simulink model "VFlexP_small"  (R2026a)
settings: Solver=ode23tb  StopTime=2  FixedStep=5e-5
model workspace (MAT data in the model file):
  DCop_DCBUCK : object (value not decoded)
  Grid_CCVSC_idx = [2; 3; 4; 5; 6; 7; 8; 9; 10; 11; 12]
  Grid_CCVSCs = 1
  Grid_CCVSCs_buses = 1
  Grid_CCVSCs_toM = [0 1 0 0 0 0 0 0 0 0 0 0 ... (781 elements, 71x11)]
  Grid_C_Lines = 0
  Grid_Cbuses = [0.00666666666667 0.00666666666667]
  Grid_DC : object (value not decoded)
  Grid_DCop_DCBUCK : object (value not decoded)
  Grid_DCop_DC_PES : object (value not decoded)
  Grid_DFIGs = 1
  Grid_DFIGs_buses = 1
  Grid_DGs : string (value not decoded)
  Grid_From_buses = 1
  Grid_GFls = 1
  Grid_GFls_buses = 1
  Grid_GFr_idx = 1
  Grid_GFrs = 1
  Grid_GFrs_buses = 1
  Grid_GFrs_toM = [1; 0]
  Grid_IG_idx = 1
  Grid_IGs = 1
  Grid_IGs_buses = 1
  Grid_IGs_toM = [1; 0; 0]
  Grid_L_Lines = 0.05
  Grid_L_Loads = [0 0]
  Grid_Lines_fromM : object (value not decoded)
  Grid_Lines_toM : object (value not decoded)
  Grid_Load_buses = [1; 2]
  Grid_Load_busesDC = []
  Grid_MSGs = 1
  Grid_MSGs_buses = 1
  Grid_Nbuses = 2
  Grid_PQ_gen = 3
  Grid_Ploads = [0.0075 0.0075]
  Grid_PloadsDC = []
  Grid_Ps_lf = 0.51232912
  Grid_Qloads = [0 0]
  Grid_Qs_lf = -0.00723209333333
  Grid_R_Lines = 0.005
  Grid_R_Loads = [2 2]
  Grid_R_Loads_DC = 0
  Grid_Rcf = [150 150]
  Grid_SCs = 1
  Grid_SCs_buses = 1
  Grid_SG_idx = 1
  Grid_SGs = 1
  Grid_SGs_buses = 1
  Grid_SGs_toM = [1; 0]
  Grid_To_buses = 2
  Grid_VCVSC_idx = [1; 2; 3; 4; 5; 6; 7; 8; 9; 10; 11; 12]
  Grid_VCVSCs = 1
  Grid_VCVSCs_buses = [1; 2; 3; 6; 8; 9; 12; 58; 59; 60; 63; 65]
  Grid_VCVSCs_toM = [1 0 0 0 0 0 0 0 0 0 0 0 ... (852 elements, 71x12)]
  Grid_VSM_idx = 2
  Grid_VSMs = 1
  Grid_VSMs_buses = 1
  Grid_VSMs_toM = [0; 1]
  Grid_admitt_matrix = [2.15353135314-19.7953135314i  -1.9801980198+19.801980198i; -1.9801980198+19.801980198i  2.15353135314-19.7953135314i]
  Grid_admitt_matrix_noloads = [1.98686468647-19.7953135314i  -1.9801980198+19.801980198i; -1.9801980198+19.801980198i  1.98686468647-19.7953135314i]
  Grid_bus = [1; 2]
  Grid_busDC_complexity = 1
  Grid_busDC_complexity_PF = 2
  Grid_bus_complexity = [1 1]
  Grid_bus_complexity_PF = [1 1]
  Grid_buses_lf = 1
  Grid_conductance_matrix = 0.00666666666667
  Grid_conductance_matrix_noloads = 0.00666666666667
  Grid_fref : object (value not decoded)
  Grid_gen_static_params : mBase (value not decoded)
  Grid_iPs_lf = 1.95187031336
  Grid_iQs_lf = -138.272551792
  Grid_iadmitt_matrix = [2.88165849328-0.0982918688642i  2.87905051706-0.123273862303i; 2.87905051706-0.123273862303i  2.88165849328-0.0982918688642i]
  Grid_iadmitt_matrix_noloads = [37.5012524798-37.4874983544i  37.4987475202-37.5125016456i; 37.4987475202-37.5125016456i  37.5012524798-37.4874983544i]
  Grid_iconductance_matrix = 150
  Grid_iconductance_matrix_noloads = 150
  Grid_init_OK_bool = 1
  Grid_intconv_PF : object (value not decoded)
  Grid_lf_op : op_report (value not decoded)
  Grid_lineDC_complexity = []
  Grid_lineDC_complexity_PF = []
  Grid_line_complexity = 1
  Grid_line_complexity_PF = 3
  Grid_loadDC_complexity = []
  Grid_loadDC_complexity_PF = []
  Grid_load_complexity = [3 3]
  Grid_load_complexity_PF = [4 4]
  Grid_opDC_CCVSC : object (value not decoded)
  Grid_opDC_VSM : object (value not decoded)
  Grid_opGFr : object (value not decoded)
  Grid_opVCVSC : object (value not decoded)
  Grid_op_CCVSC : object (value not decoded)
  Grid_op_IG : object (value not decoded)
  Grid_op_SG : object (value not decoded)
  Grid_op_VSM : object (value not decoded)
  Grid_shift_lines = 0
  Grid_tap_lines = 1
  Grid_v_buses_mod = [1 1]
  LinsysParamChangeStruct : Param1 (value not decoded)
  Lline = 0.01
  Rline = 1e-05
  linsys : object (value not decoded)
values from neighbouring files (symbols this model uses):
  block_idx = evalin(mdlWks, [bvarname Generators{i} '_idx'])    [fun_init_units_callback.m]
  Fb = areas    [fun_MATPOWER_to_Excel.m]
  Fi = evalin('base', get_param(block, 'Fi'))    [fun_init_GFr.m]    (also in fun_init_intconv_DC_VSM.m)
  Lf = evalin('base', get_param(block, 'Lf'))    [fun_init_GFr.m]    (also in fun_init_intconv_DC_VSM.m)
  Rf = evalin('base', get_param(block, 'Rf'))    [fun_init_GFr.m]    (also in fun_init_intconv_DC_VSM.m)
symbols that are objects in the model workspace (value not decoded): Grid_DCop_DC_PES, Grid_DCop_DCBUCK, Grid_op_CCVSC, Grid_op_IG, Grid_op_SG, Grid_op_VSM, Grid_opDC_CCVSC, Grid_opDC_VSM, Grid_opGFr, Grid_opVCVSC
undefined symbols (not defined in the file or in its folder): block_buses_DC, CCVSC_idx, Cf, costs, costs2, DFIGs_nodes, DiscIntNeverNeededParam, entity, From_nodes, grid_linsys, Grid_op_DFIG, Grid_op_DFIG_PQ, Grid_op_MSG, Grid_op_SC, Grid_op_VCVSC, Hv, initial_states_grid, Kic, Kiv, Kp_theta, Kp_w, Kpc, Kpv, last_send, Lc, m, Matrix_flux_to_i, mD, mp, MSGs_buses, Nbuses_DC, nq, op_VCVSC, Psche, Rc, rkq1, rkq2, SCs_buses, SCs_nodes, sec_control_structure, set_asked, set_DG_up, set_extra_satur, set_sending_cost, SGs_buses, SGs_nodes, Tf, To_nodes, VI_L, VI_R, WOF_Tf, xkq1, xkq2
libraries: simulink x1045, eeGeneralControl x12, eeTransforms x1, sl_discontinuities x1
(part 4 of 50)

== system VFlexP_small/Grid/Loadflow/Generators ==
  vd : Inport
  vq : Inport  Port=2
  Constant : Constant  Value=Ps_lf  VectorParams1D=off
  E^* : Integrator  InitialCondition=ones(1, length(buses_lf))  UpperSaturationLimit=1.2  LowerSaturationLimit=0.8
  Gain : Gain  Gain=double(PQ_gen==1)
  Gain1 : Gain  Gain=-1
  Gain10 : Gain  Gain=1e-3
  Gain11 : Gain  Gain=double(PQ_gen==3)
  Gain12 : Gain  Gain=double(PQ_gen~=3)
  Gain2 : Gain  Gain=double(PQ_gen~=1)
  Gain3 : Gain
  Gain4 : Gain
  Gain5 : Gain  Gain=double(PQ_gen==1)
  Gain6 : Gain  Gain=2*pi*50
  Gain7 : Gain  Gain=double(PQ_gen~=1)
  Gain8 : Gain  Gain=-1
  Gain9 : Gain  Gain=1e-3
  Gen_To : MATLAB Function  TreatAsAtomicUnit=on
  Gen_To1 : MATLAB Function  TreatAsAtomicUnit=on
  One1 : Constant  Value=Qs_lf  VectorParams1D=off  OutDataTypeStr=Inherit: Inherit via back propagation
  One3 : Constant  Value=v_buses_mod(buses_lf)  VectorParams1D=off  OutDataTypeStr=Inherit: Inherit via back propagation
  P : Gain  Gain=iPs_lf
  PC : Subsystem
  Q : Gain  Gain=iQs_lf
  RL out : Subsystem  Variant=on  VariantControlMode=label  LabelModeActiveChoice=dynamic  mask{dynamic=Dynamic, R=0.01, L=0.1, fbase=50}
      mask prompts: dynamic "Dynamic behavior"; R "Series resistance (p.u.)"; L "Inductance (p.u.)"; fbase "Base frequency (Hz)"
      mask init:
      | omegab = 2*pi*fbase;
      | invL = 1./L;
      | vssBlk = gcb;
      | switch dynamic
      |     case "Static"
      |         set_param(vssBlk, 'LabelModeActiveChoice', 'static');
      |     case "Dynamic"
      |         set_param(vssBlk, 'LabelModeActiveChoice', 'dynamic');
      |     case "Static omega"
      |         set_param(vssBlk, 'LabelModeActiveChoice', 'static_omega');
      | end
      mask TypeOptions dynamic: Static | Dynamic | Static omega
  Real-Imag to Complex : RealImagToComplex
  Reference frame transform1 : Subsystem
  Reference frame transform2 : Subsystem
  Reference frame transform3 : Subsystem
  Sum : Sum  Inputs=|--
  Sum1 : Sum  Inputs=|+-
  Sum2 : Sum  Inputs=-+|
  Sum3 : Sum  Inputs=|++
  Sum4 : Sum  Inputs=-+|
  Sum5 : Sum  Inputs=|--
  Sum6 : Sum  Inputs=|+-
  Sum7 : Sum  Inputs=|-+
  Sum8 : Sum  Inputs=|++
  Sum9 : Sum  Inputs=|++
  Zero : Constant  Value=0  OutDataTypeStr=Inherit: Inherit via back propagation
  \omega^* : Integrator  InitialCondition=ones(1, length(buses_lf))
  frame : Integrator  InitialCondition=zeros(1, length(buses_lf))  IgnoreLimit=on
  select_vd : Selector  InputPortWidth=Nbuses  IndexOptions=Index vector (dialog)  Indices=buses_lf  OutputSizes=1
  select_vq : Selector  InputPortWidth=Nbuses  IndexOptions=Index vector (dialog)  Indices=buses_lf  OutputSizes=1
  v : ComplexToMagnitudeAngle  Output=Magnitude
  i_d : Outport
  i_q : Outport  Port=2
  wires:
  [omega] -> Sum2/2
  Sum4/1 -> Gain9/1
  [omega] -> Sum1/1  "omega"
  [P_f] -> Sum4/2
  Sum/1 -> Gain3/1
  [P_s_to_follow] -> Sum4/1
  Gain9/1 -> Sum/2
  \omega^*/1 -> PC/3(omegaref)
  [omega_ref] -> Sum1/2
  E^*/1 -> PC/4(Eref)
  [v_to_follow] -> Sum6/2
  Sum6/1 -> Sum5/1
  Sum5/1 -> Gain4/1
  Sum7/1 -> Gain10/1
  [Q_s_to_follow] -> Sum7/1
  [vod] -> Real-Imag to Complex/1
  [Q_f] -> Sum7/2
  Gain10/1 -> Sum5/2
  PC/2(Out2) -> [vodref]
  PC/1(Out1) -> [omega]
  Q/1 -> [Q_s]
  P/1 -> [P_s]
  PC/4(Q_f) -> Q/1, [Q_f]
  PC/3(P_f) -> P/1, [P_f]
  [iod] -> PC/2(iodi)
  [theta] -> Reference frame transform3/2(theta)
  select_vd/1 -> Reference frame transform2/1(in_d), RL out/2(v_out_d)
  select_vq/1 -> Reference frame transform2/3(in_q), RL out/4(v_out_q)
  [voq] -> PC/6(voq)
  Gain1/1 -> Reference frame transform1/2(theta)
  [ioq] -> PC/1(ioq)
  Reference frame transform1/1(out_d) -> [iod]
  Reference frame transform3/1(out_d) -> RL out/1(v_in_d)
  Zero/1 -> Reference frame transform3/3(in_q)
  RL out/2(iq) -> Gen_To1/1(u), Reference frame transform1/3(in_q)
  [theta] -> Gain1/1
  Reference frame transform1/2(out_q) -> [ioq]
  Gain6/1 -> frame/1
  Reference frame transform3/2(out_q) -> RL out/3(v_in_q)
  [vod] -> PC/5(vodi)
  [vodref] -> Reference frame transform3/1(in_d)
  Gen_To/1(y) -> i_d/1
  Gen_To1/1(y) -> i_q/1
  RL out/1(id) -> Gen_To/1(u), Reference frame transform1/1(in_d)
  [omega_ref] -> Sum2/1  "ref_omega"
  Sum2/1 -> Gain6/1
  vd/1 -> select_vd/1
  vq/1 -> select_vq/1
  [P_f] -> Gain11/1
  frame/1 -> [theta]
  Constant/1 -> Gain12/1
  Sum1/1 -> Sum/1
  Gain/1 -> Sum3/1
  Gain2/1 -> Sum3/2
  Sum3/1 -> [v_to_follow]
  One3/1 -> Gain2/1
  v/1 -> Gain/1, Sum6/1
  Gain7/1 -> Sum8/2
  Gain5/1 -> Sum8/1
  [Q_f] -> Gain7/1
  One1/1 -> Gain5/1
  Sum8/1 -> [Q_s_to_follow]
  Gain4/1 -> E^*/1
  Gain3/1 -> \omega^*/1
  [theta] -> Gain8/1
  Gain8/1 -> Reference frame transform2/2(theta)
  Reference frame transform2/2(out_q) -> [voq]
  Reference frame transform2/1(out_d) -> [vod]
  [voq] -> Real-Imag to Complex/2
  Real-Imag to Complex/1 -> v/1
  Sum9/1 -> [P_s_to_follow]
  Gain11/1 -> Sum9/1
  Gain12/1 -> Sum9/2

== system VFlexP_small/Grid/Loadflow/Grid ==
  note: 1) Add Subsystem or Model blocks as valid variant choices.
      | 2) You cannot connect blocks at this level. At simulation, connectivity is automatically
      | determined, based on the active variant and port name matching.
  id_in : Inport
  iq_in : Inport  Port=2
  id_out : Inport  Port=3
  iq_out : Inport  Port=4
  Dynamic : Subsystem  VariantControl=Dynamic
  Static : Subsystem  VariantControl=Static
  vd : Outport
  vq : Outport  Port=2

== system VFlexP_small/Grid/Loadflow/Loads ==
  vd : Inport
  vq : Inport  Port=2
  PQ : Subsystem  VariantControl=PQ
  Sum : Sum  Inputs=|+++++
  Sum1 : Sum  Inputs=|+++++
  dynamic : Subsystem  Commented=on  VariantControl=dynamic
  dynamic PQ : Subsystem  Commented=on  VariantControl=PQ
  static : Subsystem  Commented=on  VariantControl=static
  static omega : Subsystem  Commented=on  VariantControl=static_omega
  id : Outport
  iq : Outport  Port=2
  wires:
  dynamic/1(id) -> Sum/1
  vq/1 -> dynamic PQ/2(v_in_q), PQ/2(v_in_q), static omega/2(v_in_q), static/2(v_in_q), dynamic/2(v_in_q)
  PQ/2(iq) -> Sum1/4
  dynamic PQ/2(iq) -> Sum1/5
  vd/1 -> dynamic PQ/1(v_in_d), PQ/1(v_in_d), static omega/1(v_in_d), static/1(v_in_d), dynamic/1(v_in_d)
  static omega/1(id) -> Sum/3
  Sum/1 -> id/1  "id"
  static omega/2(iq) -> Sum1/3
  dynamic PQ/1(id) -> Sum/5
  static/2(iq) -> Sum1/2
  Sum1/1 -> iq/1  "iq"
  dynamic/2(iq) -> Sum1/1
  PQ/1(id) -> Sum/4
  static/1(id) -> Sum/2

== system VFlexP_small/Grid/Loadflow/to_all_Nodes ==
  In1 : Inport
  Assignment : Assignment  DiagnosticForDimensions=Warning  IndexOptions=Index vector (dialog)  Indices=Load_buses  OutputSizes=1
  Zero : Constant  Value=zeros(1,Nbuses)  VectorParams1D=off  OutDataTypeStr=Inherit: Inherit via back propagation
  id_out : Outport
  wires:
  Zero/1 -> Assignment/1
  In1/1 -> Assignment/2
  Assignment/1 -> id_out/1

== system VFlexP_small/Grid/Loadflow/to_all_Nodes1 ==
  In1 : Inport
  Assignment : Assignment  DiagnosticForDimensions=Warning  IndexOptions=Index vector (dialog)  Indices=Load_buses  OutputSizes=1
  Zero : Constant  Value=zeros(1,Nbuses)  VectorParams1D=off  OutDataTypeStr=Inherit: Inherit via back propagation
  iq_out : Outport
  wires:
  Assignment/1 -> iq_out/1
  In1/1 -> Assignment/2
  Zero/1 -> Assignment/1

== system VFlexP_small/Grid/Dynamic/DCAC converters/DC_CCVSC ==
  note: port number 2
  note: do not rename this block, conditions to initialise the generator from PF result are set on this block's output
  vac : Inport
  vdc : Inport  Port=2
  Abs : Abs  SaturateOnIntegerOverflow=off
  CC : Subsystem  Variant=on  VariantControlMode=label  LabelModeActiveChoice=dynamic
  Cast To Double : DataTypeConversion  OutDataTypeStr=double  SaturateOnIntegerOverflow=off  RndMeth=Floor
  Compare To Constant : simulink/Logic and Bit Operations/Compare To Constant  relop===  const=2  OutDataTypeStr=boolean
  Complex to Magnitude-Angle : ComplexToMagnitudeAngle  Output=Angle
  Constant : Constant  Value=zeros(1, length(block_buses))  VectorParams1D=off
  Constant1 : Constant  Value=dparams.alpha1  VectorParams1D=off
  Constant2 : Constant  Value=dparams.type  VectorParams1D=off
  Constant3 : Constant  Value=DC.v(block_DC_buses)  VectorParams1D=off
  Divide : Product  Inputs=*/
  For Each Subsystem : Subsystem  TreatAsAtomicUnit=on
  Gain : Gain  Gain=-1
  Gain1 : Gain  Gain=dparams.alpha2
  Gain10 : Gain  Gain=-1
  Gain2 : Gain  Gain=dparams.alpha3
  Gain5 : Gain  Gain=0.5
  Gain8 : Gain  Gain=10
  Gain9 : Gain
  Gsw : Constant  Value=dparams.Gsw.*(dparams.alpha1 == 0 & dparams.alpha2 == 0 & dparams.alpha3 == 0)  VectorParams1D=off
  I : Integrator  InitialCondition=Grid_opDC_CCVSC.P
  LPF_d : Subsystem
  LPF_q : Subsystem
  Matrix Concatenate1 : Concatenate  NumInputs=3  Mode=Multidimensional array
  One : Constant  OutDataTypeStr=Inherit: Inherit via back propagation
  P : Integrator  InitialCondition=Grid_opDC_CCVSC.P
  PC : Subsystem
      settings: PortSchema="{\"entries\":[{\"content\":{\"sides\":[{\"content\":{\"connectorIds\":[\"In1\",\"In2\",\"In3\",\"In4\"]},\"type\":\"ConnectorPlacement.EquallySpacedRectSide\",\"uuid\":\"7748ce6f-2dcc-431c-b3ea-0be9c3088b1d\"},{\"content\":{\"connectorIds\":[\"In5\",\"Out1\",\"Out2\"],\"side\":\"RIGHT\"},\"type\":\"ConnectorPlacement.EquallySpacedRectSide\",\"uuid\":\"af86fd8d-043b-4d20-8ee8-e7a977d706a8\"},{\"content\":{\"side\":\"TOP\"},\"type\":\"ConnectorPlacement.EquallySpacedRectSide\",\"uuid\":\"807e0dc6-0d59-4ea5-9557-3ccfd29c2ad0\"}]},\"type\":\"ConnectorPlacement.EquallySpacedConnector\",\"uuid\":\"c7fe00c5-0a0a-4038-b7ac-e659fb2aa4a7\"}],\"packageUris\":[\"http://schema.mathworks.com/mf0/Connector/R2020b\"],\"version\":\"1.0\"}"
  PLL : Subsystem  Variant=on  VariantControlMode=label  LabelModeActiveChoice=dynamic
  Product{,1..5,8} (7 alike) : Product
  Product6 : Product  Inputs=3
  Q : Integrator  InitialCondition=Grid_opDC_CCVSC.Q
  Real-Imag to Complex : RealImagToComplex
  Real-Imag to Complex1 : RealImagToComplex
  Reference frame transform3 : Subsystem
  Reference_frame_transform1 : Subsystem
  Scope : Scope
      settings: ActiveDisplayYMinimum=-0.01179  ActiveDisplayYMaximum=0.0098
  Scope1 : Scope
      settings: ActiveDisplayYMinimum=-0.59827  ActiveDisplayYMaximum=0.48453  DataLoggingVariableName=ScopeData2
  Selector : Selector  InputPortWidth=DC.Nbuses  IndexOptions=Index vector (dialog)  Indices=block_DC_buses  OutputSizes=1
  Selector5 : Selector  NumberOfDimensions=2  InputPortWidth=3  IndexOptions=Index vector (dialog),Index vector (dialog)  Indices=1,block_buses  OutputSizes=1,1
  Selector6 : Selector  NumberOfDimensions=2  InputPortWidth=3  IndexOptions=Index vector (dialog),Index vector (dialog)  Indices=2,block_buses  OutputSizes=1,1
  Selector7 : Selector  InputPortWidth=length(fref.ref_units)  IndexOptions=Index vector (dialog)  Indices=block_fref  OutputSizes=1
  Signal Specification1 : SignalSpecification  Dimensions=[3 length(block_buses)]
  State-Space : StateSpace  A=[]  B=[]  C=[]  D=block_DC_toM  InitialCondition=0  ParameterTunability=Optimized
  Sum : Sum  Inputs=|++
  Sum1 : Sum  Inputs=|-+
  Sum2 : Sum  Inputs=|++
  Sum4 : Sum  Inputs=+|+|+
  Sum5 : Sum  Inputs=+|+|+
  Sum6 : Sum  Inputs=|++
  Sum7 : Sum  Inputs=|+-
  Switch : Switch  Criteria=u2 > Threshold  SaturateOnIntegerOverflow=off  InputSameDT=off
  Terminator{,3..5} (4 alike) : Terminator
  Transpose : Math  Operator=transpose
  Transpose1 : Math  Operator=transpose
  connect : Subsystem
  connect1 : Subsystem
      settings: PortSchema="{\"entries\":[{\"content\":{\"sides\":[{\"content\":{\"connectorIds\":[\"In1\",\"In2\"]},\"type\":\"ConnectorPlacement.EquallySpacedRectSide\",\"uuid\":\"6197940c-2174-4524-96b1-99ee20c84056\"},{\"content\":{\"connectorIds\":[\"Out1\",\"Out2\"],\"side\":\"RIGHT\"},\"type\":\"ConnectorPlacement.EquallySpacedRectSide\",\"uuid\":\"9096a550-ff71-4818-a7e7-327a4860b088\"},{\"content\":{\"connectorIds\":[\"In3\"],\"side\":\"TOP\"},\"type\":\"ConnectorPlacement.EquallySpacedRectSide\",\"uuid\":\"d804310e-982f-4fb4-ab62-6be4f27f3ef7\"}]},\"type\":\"ConnectorPlacement.EquallySpacedConnector\",\"uuid\":\"3c08874d-8366-4035-b771-5fa3fbbe507b\"}],\"packageUris\":[\"http://schema.mathworks.com/mf0/Connector/R2020b\"],\"version\":\"1.0\"}"
  trim_output : Subsystem
  iac : Outport
  idc : Outport  Port=2
  wires:
  vac/1 -> Selector5/1, Selector6/1
  Selector6/1 -> [vqout], trim_output/4(vq)
  Selector5/1 -> [vdout], trim_output/3(vd)
  trim_output/4(Out4) -> Terminator5/1
  trim_output/2(Out2) -> Terminator3/1
  trim_output/3(Out3) -> Terminator4/1
  trim_output/1(Out1) -> Terminator/1
  For Each Subsystem/1(Out1) -> iac/1
  Constant/1 -> Matrix Concatenate1/3
  Signal Specification1/1 -> For Each Subsystem/1(In1)
  Matrix Concatenate1/1 -> Signal Specification1/1
  [v_q_PCC] -> Reference frame transform3/3(in_q), Real-Imag to Complex/2  "voq"
  [v_d_PCC] -> Reference frame transform3/1(in_d), Real-Imag to Complex/1  "vod"
  connect/2(iq_real) -> Matrix Concatenate1/2, trim_output/2(iq), [ioq]
  connect/1(id_real) -> Matrix Concatenate1/1, trim_output/1(id), [iod]
  One/1 -> connect/3(connect), connect1/3(connect)
  Cast To Double/1 -> [connected]
  Reference_frame_transform1/1(dout) -> connect/1(id)
  Reference_frame_transform1/2(qout) -> connect/2(iq)
  PLL/2(omega_point) -> [omega], CC/5(omega)  "\\omega CCVSC"
  Complex to Magnitude-Angle/1 -> [voutangle]
  Real-Imag to Complex/1 -> Complex to Magnitude-Angle/1
  [vod] -> CC/3(vod), PC/1(vodi)
  [voq] -> CC/4(voq), PC/2(voq)
  Reference frame transform3/1(out_d) -> [vod]  "v CCVSC"
  [v_q_PCC] -> Product1/1  "voq"
  Sum/1 -> LPF_d/1(In1)
  Sum1/1 -> LPF_q/1(In1)
  [iod] -> Product3/2  "iod"
  [ioq] -> Product2/2  "ioq"
  Product2/1 -> Sum1/1
  Product1/1 -> Sum/2
  Product3/1 -> Sum1/2
  Product/1 -> Sum/1
  LPF_d/1(Out1) -> Scope/1, [P_s]
  LPF_q/1(Out1) -> Scope1/1, [Q_s]
  [v_d_PCC] -> Product/1  "vod"
  [iod] -> Product/2  "iod"
  [ioq] -> Product1/2  "ioq"
  [v_d_PCC] -> Product2/1  "vod"
  [v_q_PCC] -> Product3/1  "voq"
  PC/1(Output) -> CC/1(idref)  "iod"
  PC/2(Output1) -> CC/2(iqref)  "ioq"
  [theta] -> Gain/1
  Gain/1 -> Reference frame transform3/2(theta)
  [theta] -> Reference_frame_transform1/3(theta)
  [voq] -> PLL/2(vq)
  [omega_ref] -> Selector7/1
  PLL/1(theta) -> [theta]
  Reference frame transform3/2(out_q) -> [voq]
  connect/3(connected) -> Cast To Double/1
  Q/1 -> PC/4(vodi2)
  [voutangle] -> PLL/1(voutangle)
  Product4/1 -> Sum2/1
  Product5/1 -> Sum2/2
  connect1/2(iq_real) -> Product5/2, Real-Imag to Complex1/2  "ioq"
  connect1/1(id_real) -> Real-Imag to Complex1/1, Product4/2  "iod"
  CC/3(vid) -> Product4/1
  CC/4(viq) -> Product5/1
  Real-Imag to Complex1/1 -> Abs/1
  Constant1/1 -> Sum4/3
  Gain1/1 -> Sum4/2
  Product8/1 -> Gain2/1
  Gain2/1 -> Sum4/1
  Sum5/1 -> Gain10/1  "Pdc"
  Divide/1 -> Transpose/1  "iDC"
  [vdout] -> [v_d_PCC]
  [vqout] -> [v_q_PCC]
  P/1 -> Switch/3
  Switch/1 -> PC/3(vodi1)
  Constant2/1 -> Compare To Constant/1
  Gain5/1 -> Sum6/1
  I/1 -> Sum6/2
  Gain8/1 -> I/1
  Sum6/1 -> Switch/1
  Constant3/1 -> Sum7/2
  Gain9/1 -> Gain8/1, Gain5/1
  CC/1(idiref) -> connect1/1(id), Reference_frame_transform1/1(din)
  CC/2(iqiref) -> Reference_frame_transform1/2(qin), connect1/2(iq)  "ioq"
  Sum7/1 -> Gain9/1
  Compare To Constant/1 -> Switch/2
  Sum2/1 -> Sum5/2
  Gain10/1 -> Divide/1
  Product6/1 -> Sum5/3
  Abs/1 -> Product8/2, Product8/1, Gain1/1
  Sum4/1 -> Sum5/1
  Gsw/1 -> Product6/1
  State-Space/1 -> Transpose1/1
  Transpose/1 -> State-Space/1
  [vDC] -> Sum7/1
  Selector7/1 -> PC/5(omega), PLL/3(omega)
  Transpose1/1 -> idc/1
  Selector/1 -> Product6/3, Product6/2, [vDC], Divide/2
  vdc/1 -> Selector/1

== system VFlexP_small/Grid/Dynamic/DCAC converters/DC_VCVSC ==
  note: port number 2
  note: do not rename this block, conditions to initialise the generator from PF result are set on this block's output
  vac : Inport
  vdc : Inport  Port=2
  AND : Logic  IconShape=distinctive  AllPortsSameDT=off  OutDataTypeStr=boolean
  AND1 : Logic  Inputs=3  IconShape=distinctive  AllPortsSameDT=off  OutDataTypeStr=boolean
  AND2 : Logic  IconShape=distinctive  AllPortsSameDT=off  OutDataTypeStr=boolean
  Abs{,1..3} (4 alike) : Abs  ZeroCross=off  SaturateOnIntegerOverflow=off
  Atan2 : Trigonometry  Operator=atan2
  Cast To Double2 : DataTypeConversion  OutDataTypeStr=double  SaturateOnIntegerOverflow=off  RndMeth=Floor
  Compare To Constant : simulink/Logic and Bit Operations/Compare To Constant  relop=<=  const=0.001  OutDataTypeStr=boolean  ZeroCross=off
  Compare To Constant1 : simulink/Logic and Bit Operations/Compare To Constant  relop=<=  const=0.01  OutDataTypeStr=boolean  ZeroCross=off
  Compare To Constant2 : simulink/Logic and Bit Operations/Compare To Constant  relop=<=  const=0.2  OutDataTypeStr=boolean  ZeroCross=off
  Compare To Constant3 : simulink/Logic and Bit Operations/Compare To Constant  relop=>  const=4  OutDataTypeStr=boolean  ZeroCross=off
  Complex to Real-Imag : ComplexToRealImag
  Conjugate : Math  Operator=conj  SignedPower=on  RndMeth=Zero
  Constant : Constant  Value=zeros(1, length(block_buses))  VectorParams1D=off
  Constant1 : Constant  Value=5*ones(1,length(block_idx))  VectorParams1D=off
  Constant2 : Constant  Value=zeros(1,length(block_idx))  VectorParams1D=off
  For Each Subsystem : Subsystem  TreatAsAtomicUnit=on
  Gain1 : Gain  Gain=-1
  Gain2 : Gain  Gain=-1
  Gain6 : Gain  Gain=2*pi*fb
  Gen_To_DC : MATLAB Function  TreatAsAtomicUnit=on
  Integrator : Integrator  ExternalReset=falling  InitialConditionSource=external  InitialCondition=Grid_op_VCVSC.States(1,:)
  Integrator1 : Integrator  InitialCondition=Grid_op_VCVSC.States(2,:)
  LPF : Subsystem  Commented=through
  LPF1 : Subsystem  Commented=through
  LPF2 : Subsystem
  LPF3 : Subsystem
  Matrix Concatenate1 : Concatenate  NumInputs=3  Mode=Multidimensional array
  Memory2 : Memory  InitialCondition=1
  NOT1 : Logic  Operator=NOT  IconShape=distinctive  AllPortsSameDT=off  OutDataTypeStr=boolean
  OR : Logic  Operator=OR  Inputs=3  IconShape=distinctive  AllPortsSameDT=off  OutDataTypeStr=boolean
  PC : Subsystem  mask(PC_VCVSC){Tf=Tf, mp=mp, nq=nq}
      mask prompts: Tf "Low-pass filter time constant (s)"; mp "Droop coefficient mp"; nq "Droop coefficient nq"
      mask help: Power controller of a grid-forming converter, including the droop control and low-pass filters for the power measurements.
      mask init:
      | if all(Tf ~= 0)
      |     iTf = 1./Tf;
      |     set_param([gcb '/LPF_P'],'Commented','off')
      |     set_param([gcb '/LPF_Q'],'Commented','off')
      | else
      |     set_param([gcb '/LPF_P'],'Commented','through')
      |     set_param([gcb '/LPF_Q'],'Commented','through')
      | end
  PI : Subsystem
  PI1 : Subsystem
  Product : Product
  Product1 : Product  OutDataTypeStr=double
  Product2 : Product  OutDataTypeStr=double
  RL out : Subsystem  Variant=on  VariantControlMode=label  LabelModeActiveChoice=dynamic  mask{dynamic=Dynamic, R=R_out, L=L_out, fbase=50}
      mask prompts: dynamic "Dynamic behavior"; R "Series resistance (p.u.)"; L "Inductance (p.u.)"; fbase "Base frequency (Hz)"
      mask init: same as VFlexP_small/Grid/Loadflow/Generators/RL out
      mask TypeOptions dynamic: Static | Dynamic | Static omega
  Real-Imag to Complex : RealImagToComplex
  Real-Imag to Complex1 : RealImagToComplex
  Reference frame transform1 : Subsystem
  Reference frame transform2 : Subsystem
  Reference frame transform3 : Subsystem
  Selector5 : Selector  NumberOfDimensions=2  InputPortWidth=3  IndexOptions=Index vector (dialog),Index vector (dialog)  Indices=1,block_buses  OutputSizes=1,1
  Selector6 : Selector  NumberOfDimensions=2  InputPortWidth=3  IndexOptions=Index vector (dialog),Index vector (dialog)  Indices=2,block_buses  OutputSizes=1,1
  Signal Specification1 : SignalSpecification  Dimensions=[3 length(block_buses)]
  Step : Step  Time=0.01  SampleTime=0  VectorParams1D=off  ZeroCross=off
  Sum1 : Sum  Inputs=|++
  Sum11 : Sum  Inputs=|++
  Sum12 : Sum  Inputs=|++
  Sum2 : Sum  Inputs=-+|
  Sum3 : Sum  Inputs=|+-
  Sum8 : Sum  Inputs=++|
  Switch : Switch  Criteria=u2 > Threshold  SaturateOnIntegerOverflow=off  InputSameDT=off
  Switch2 : Switch  Criteria=u2 > Threshold  SaturateOnIntegerOverflow=off  InputSameDT=off
  Switch3 : Switch  Criteria=u2 > Threshold  SaturateOnIntegerOverflow=off  InputSameDT=off
  Terminator{,1..5} (6 alike) : Terminator
  VCC : Subsystem  Variant=on  VariantControlMode=label  LabelModeActiveChoice=static
  VI : Subsystem  Commented=on  mask{L=VI_L, R=VI_R, Tf=WOF_Tf}
      mask prompts: L "Inductance (pu)"; R "Resistance (pu)"; Tf "WOF time constant (s)"
      mask init:
      | if all(Tf ~= 0)
      |     iTf = 1./Tf;
      |     set_param([gcb '/WOF_d'],'Commented','off')
      |     set_param([gcb '/WOF_q'],'Commented','off')
      | else
      |     set_param([gcb '/WOF_d'],'Commented','through')
      |     set_param([gcb '/WOF_q'],'Commented','through')
      | end
  Zero : Constant  Value=0  OutDataTypeStr=Inherit: Inherit via back propagation
  connect : Subsystem
  frame : Integrator  InitialCondition=Grid_op_VCVSC.States(19,:)  IgnoreLimit=on
  trim_output : Subsystem
  vod : Sum  Inputs=++|
  iac : Outport
  idc : Outport  Port=2
  wires:
  LPF3/1(Out1) -> PC/4(Eref)
  LPF2/1(Out1) -> PC/3(omegaref)
  [connect] -> AND2/2
  Compare To Constant3/1 -> connect/3(connect)
  Integrator1/1 -> Sum1/2
  [v_to_follow] -> Sum1/1
  [Q_s_to_follow] -> PC/8(Qsp)
  [P_s_to_follow] -> PC/7(Psp)
  Switch2/1 -> LPF3/1(In1)
  Switch3/1 -> LPF2/1(In1)
  Sum11/1 -> Switch3/3
  PI1/1(Out1) -> Sum11/1
  PI/1(Out1) -> Sum12/1
  [connected] -> Switch3/2, Switch2/2
  [omega_to_follow] -> Switch3/1, Sum11/2
  Sum1/1 -> Sum12/2, Switch2/1
  Sum12/1 -> Switch2/3
  VCC/2(viqref) -> Reference frame transform3/3(in_q), [voq]
  VCC/1(vidref) -> Reference frame transform3/1(in_d), [vod]
  Switch/1 -> Integrator/3
  Cast To Double2/1 -> Integrator/1
  AND1/1 -> Integrator/2, Cast To Double2/1
  [safe_to_connect] -> AND1/3
  Constant1/1 -> Switch/3
  Step/1 -> AND1/1, Switch/2
  Constant2/1 -> Switch/1
  Integrator/1 -> Compare To Constant3/1
  [connect] -> AND1/2
  AND2/1 -> Product2/1, Product1/1
  [connected] -> NOT1/1
  NOT1/1 -> AND2/1
  Selector5/1 -> trim_output/3(vd), [vdout]
  Selector6/1 -> trim_output/4(vq), [vqout]
  vac/1 -> Selector5/1, Selector6/1
  trim_output/4(Out4) -> Terminator5/1
  trim_output/3(Out3) -> Terminator4/1
  trim_output/2(Out2) -> Terminator3/1
  trim_output/1(Out1) -> Terminator/1
  [v_q_PCC] -> PC/6(voq)
  [v_d_PCC] -> PC/5(vodi)
  Signal Specification1/1 -> For Each Subsystem/1(In1)
  For Each Subsystem/1(Out1) -> iac/1
  Constant/1 -> Matrix Concatenate1/3
  Matrix Concatenate1/1 -> Signal Specification1/1
  [vdout] -> Reference frame transform2/1(in_d), RL out/2(v_out_d)
  LPF1/1(Out1) -> [v_q_PCC]
  LPF/1(Out1) -> [v_d_PCC]
  [vqout] -> RL out/4(v_out_q), Reference frame transform2/3(in_q)
  Memory2/1 -> [safe_to_connect]
  [connected] -> OR/3
  Compare To Constant2/1 -> OR/2
  OR/1 -> Memory2/1
  AND/1 -> OR/1
  Compare To Constant1/1 -> AND/1
  Abs3/1 -> Compare To Constant1/1
  Compare To Constant/1 -> AND/2
  Abs2/1 -> Compare To Constant/1
  Abs1/1 -> Sum3/2, Compare To Constant2/1
  Atan2/1 -> Product2/2, Abs3/1
  Product2/1 -> PI1/1(In1)
  Product1/1 -> PI/1(In1)
  Sum3/1 -> Product1/2, Abs2/1
  Abs/1 -> Sum3/1
  Complex to Real-Imag/1 -> Atan2/2
  Complex to Real-Imag/2 -> Atan2/1
  Product/1 -> Complex to Real-Imag/1
  Conjugate/1 -> Product/2
  Real-Imag to Complex/1 -> Product/1, Abs/1
  Real-Imag to Complex1/1 -> Conjugate/1, Abs1/1
  [voq] -> Real-Imag to Complex1/2
  [vod] -> Real-Imag to Complex1/1
  [v_q_PCC] -> Real-Imag to Complex/2
  [v_d_PCC] -> Real-Imag to Complex/1
  Reference frame transform2/2(out_q) -> LPF1/1(In1)
  Reference frame transform2/1(out_d) -> LPF/1(In1)
  RL out/4(v_outq) -> Terminator2/1
  RL out/3(v_outd) -> Terminator1/1
  connect/2(iq_real) -> Reference frame transform1/3(in_q), Matrix Concatenate1/2, trim_output/2(iq)
  connect/1(id_real) -> Reference frame transform1/1(in_d), Matrix Concatenate1/1, trim_output/1(id)
  VI/2(vq) -> Sum8/1
  VI/1(vd) -> vod/1
  Reference frame transform1/1(out_d) -> [iod]
  RL out/2(iq) -> connect/2(iq)
  Reference frame transform3/2(out_q) -> RL out/3(v_in_q)
  Reference frame transform3/1(out_d) -> RL out/1(v_in_d)
  Reference frame transform1/2(out_q) -> [ioq]
  [ioq] -> PC/1(ioq)
  [iod] -> PC/2(iodi)
  PC/2(Out2) -> [vodref]
  PC/1(Out1) -> [omega]
  [theta] -> Reference frame transform3/2(theta)
  [omega] -> VCC/5(omega)
  [vodref] -> vod/2
  Zero/1 -> Sum8/2
  [iod] -> VCC/3(iod)
  [ioq] -> VCC/4(ioq)
  Gain1/1 -> Reference frame transform1/2(theta)
  [theta] -> Gain1/1
  RL out/1(id) -> connect/1(id)
  Sum2/1 -> Gain6/1
  [omega_ref] -> Sum2/1  "ref_omega"
  [omega] -> Sum2/2  "omega"
  connect/3(connected) -> [connected]
  PC/3(P_f) -> [P_f], [P_s]
  PC/4(Q_f) -> [Q_f], [Q_s]
  frame/1 -> [theta]
  Gain6/1 -> frame/1
  [theta] -> Gain2/1
  Gain2/1 -> Reference frame transform2/2(theta)
  [iod] -> VI/1(id)
  [ioq] -> VI/2(iq)
  [omega] -> VI/3(omega)
  vod/1 -> VCC/1(vodref)
  Sum8/1 -> VCC/2(voqref)

== system VFlexP_small/Grid/Dynamic/DCAC converters/DC_VSM ==
  note: do not rename this block, conditions to initialise the generator from PF result are set on this block's output
  note: port number 2
  vac : Inport
  vdc : Inport  Port=2
  Abs4 : Abs  SaturateOnIntegerOverflow=off
  Active power (pu) : Scope  NumInputPorts=2
      settings: ActiveDisplayYMinimum=0.451710825505785  ActiveDisplayYMaximum=0.62051523001208286  DataLoggingVariableName=ScopeData13
  Complex to Magnitude-Angle : ComplexToMagnitudeAngle
  Constant : Constant  Value=zeros(1, length(block_buses))  VectorParams1D=off
  Constant1 : Constant  Value=dparams.alpha1  VectorParams1D=off
  Constant2 : Constant  Value=Grid_opDC_VSM.P
  Constant3 : Constant  Value=Grid_opDC_VSM.Q
  Constant4 : Constant  Value=0.5
  Constant5 : Constant
  Constant6 : Constant  Value=0.3425
  Dead Zone : DeadZone  LowerValue=-0.2  UpperValue=0.2
  Derivative : Derivative
  Divide : Product  Inputs=*/
  For Each Subsystem : Subsystem  TreatAsAtomicUnit=on
  From File : FromFile  FileName=u2_combined.mat  SampleTime=0
  From File1 : FromFile  FileName=p_out_combined.mat  SampleTime=0
  Gain : Gain  Gain=180
  Gain{1..2,10,17} (4 alike) : Gain  Gain=-1
  Gain11 : Gain  Gain=0.00015
  Gain12 : Gain  Gain=0.57
  Gain14 : Gain  Gain=20
  Gain15 : Gain  Gain=100
  Gain16 : Gain  Gain=1/(2*pi*50)
  Gain18 : Gain  Gain=2*pi*50
  Gain3 : Gain  Gain=dparams.alpha2
  Gain4 : Gain  Gain=dparams.alpha3
  Gain5 : Gain  Gain=Kp_theta
  Gain6 : Gain  Gain=Kp_w
  Gain7 : Gain  Gain=2*pi*fb
  Gain8 : Gain  Gain=0.066
  Gsw : Constant  Value=dparams.Gsw.*(dparams.alpha1 == 0 & dparams.alpha2 == 0 & dparams.alpha3 == 0)  VectorParams1D=off
  Integrator1 : Integrator
  Integrator2 : Integrator
  Inverse Park Transform : eeTransforms/Inverse Park Transform  AxisAlignment=Q-axis  PowerInvariant=off
      settings: LibrarySourceBlock=|
      | ee_sl_lib/Mathematical
      | Transforms/Inverse
      | Park Transform
  LPF : Subsystem  Commented=through
  LPF1 : Subsystem  Commented=through
  LPF2 : Subsystem
  LPF_1 : Subsystem
  LPF_2 : Subsystem
  LPF_Pi : Scope  NumInputPorts=2
      settings: ActiveDisplayYMinimum=-0.18032060952587592  ActiveDisplayYMaximum=0.032176801057402428  DataLoggingVariableName=ScopeData10
  Matrix Concatenate1 : Concatenate  NumInputs=3  Mode=Multidimensional array
  Mux{,1,3..4} (4 alike) : Mux  Inputs=2
  Mux2 : Mux  Inputs=3
  One : Constant  OutDataTypeStr=Inherit: Inherit via back propagation
  One1 : Constant  OutDataTypeStr=Inherit: Inherit via back propagation
  One2 : Constant  OutDataTypeStr=Inherit: Inherit via back propagation
  PC : Subsystem  mask(PC_VCVSC){Tf=0.01, mp=0.01, nq=0.01}
      mask prompts: Tf "Low-pass filter time constant (s)"; mp "Droop coefficient mp"; nq "Droop coefficient nq"
      mask help: Power controller of a grid-forming converter, including the droop control and low-pass filters for the power measurements.
      mask init: same as VFlexP_small/Grid/Dynamic/DCAC converters/DC_VCVSC/PC
  PLL : Subsystem
  Product{,4..5,8} (4 alike) : Product
  Product6 : Product  Inputs=3
  RL out : Subsystem  Variant=on  VariantControlMode=label  LabelModeActiveChoice=dynamic  mask{dynamic=Dynamic, R=dparams.Rf, L=dparams.Lf, fbase=50}
      mask prompts: dynamic "Dynamic behavior"; R "Series resistance (p.u.)"; L "Inductance (p.u.)"; fbase "Base frequency (Hz)"
      mask init: same as VFlexP_small/Grid/Loadflow/Generators/RL out
      mask TypeOptions dynamic: Static | Dynamic | Static omega
  Real-Imag to Complex : RealImagToComplex
  Real-Imag to Complex2 : RealImagToComplex
  Reference frame transform1 : Subsystem
  Reference frame transform2 : Subsystem
  Reference frame transform3 : Subsystem
  Reference frame transform4 : Subsystem
      settings: PortSchema="{\"entries\":[{\"content\":{\"sides\":[{\"content\":{\"connectorIds\":[\"In1\",\"In2\"]},\"type\":\"ConnectorPlacement.EquallySpacedRectSide\",\"uuid\":\"2587aae9-c00d-40c4-a574-3c07a0e9f6d0\"},{\"content\":{\"connectorIds\":[\"Out1\",\"Out2\",\"In3\"],\"side\":\"RIGHT\"},\"type\":\"ConnectorPlacement.EquallySpacedRectSide\",\"uuid\":\"821c99fc-5155-4d87-994b-2bceacdbfd1f\"},{\"content\":{\"side\":\"TOP\"},\"type\":\"ConnectorPlacement.EquallySpacedRectSide\",\"uuid\":\"7906fa13-ffc3-450b-b804-9b291a4ef523\"}]},\"type\":\"ConnectorPlacement.EquallySpacedConnector\",\"uuid\":\"1e7d1263-3ba5-4f7a-8418-30f696cdbf3e\"}],\"packageUris\":[\"http://schema.mathworks.com/mf0/Connector/R2020b\"],\"version\":\"1.0\"}"
  Scope : Scope  NumInputPorts=2
      settings: ActiveDisplayYMinimum=0.95813  ActiveDisplayYMaximum=1.0211
  Scope1 : Scope
      settings: ActiveDisplayYMinimum=-5.1734  ActiveDisplayYMaximum=7.213  DataLoggingVariableName=ScopeData2
  Scope2 : Scope
      settings: ActiveDisplayYMinimum=-6.983  ActiveDisplayYMaximum=8.3015  DataLoggingVariableName=ScopeData3
  Scope3 : Scope
      settings: ActiveDisplayYMinimum=-1.3624  ActiveDisplayYMaximum=1.2686  DataLoggingVariableName=ScopeData4
  Selector : Selector  InputPortWidth=DC.Nbuses  IndexOptions=Index vector (dialog)  Indices=block_DC_buses  OutputSizes=1
  Selector5 : Selector  NumberOfDimensions=2  InputPortWidth=3  IndexOptions=Index vector (dialog),Index vector (dialog)  Indices=1,block_buses  OutputSizes=1,1
  Selector6 : Selector  NumberOfDimensions=2  InputPortWidth=3  IndexOptions=Index vector (dialog),Index vector (dialog)  Indices=2,block_buses  OutputSizes=1,1
  Signal Specification1 : SignalSpecification  Dimensions=[3 length(block_buses)]
  Square : Math  Operator=square
  Square1 : Math  Operator=square
  State-Space : StateSpace  A=[]  B=[]  C=[]  D=block_DC_toM  InitialCondition=0  ParameterTunability=Optimized
  Step : Step  Time=0.05  SampleTime=0
  Step1 : Step  Time=0.1  InitialValue=-0.501  FinalValue=-0.1-0.501  SampleTime=0
  Step3 : Step  Time=22  FinalValue=0.1  SampleTime=0
  Sum{,1,4,7,9..10,12..13,15..16} (10 alike) : Sum  Inputs=|++
  Sum11 : Sum  Inputs=|+-
  Sum14 : Sum  Inputs=|+-
  Sum2 : Sum  Inputs=-+|
  Sum3 : Sum  Inputs=|+-
  Sum5 : Sum  Inputs=+|+|+
  Sum6 : Sum  Inputs=+|+|+
  Sum8 : Sum  Inputs=++|
  Terminator{,1..5} (6 alike) : Terminator
  To File : ToFile  Filename=Pi_VSM  MatrixName=Pi_VSM  SaveFormat=Timeseries
  To Workspace : ToWorkspace  VariableName=u2  SaveFormat=Structure With Time  SampleTime=-1
  To Workspace1 : ToWorkspace  VariableName=Pout  SaveFormat=Structure With Time  SampleTime=-1
  To Workspace2 : ToWorkspace  VariableName=Poutf  SaveFormat=Structure With Time  SampleTime=-1
  Transpose : Math  Operator=transpose
  Transpose1 : Math  Operator=transpose
  VCC : Subsystem  Variant=on  VariantControlMode=label  LabelModeActiveChoice=dynamic_limiting_P
      settings: PortSchema="{\"entries\":[{\"content\":{\"sides\":[{\"content\":{\"connectorIds\":[\"In1\",\"In2\",\"In3\",\"In4\",\"In5\"]},\"type\":\"ConnectorPlacement.EquallySpacedRectSide\",\"uuid\":\"7244c354-1494-46e2-b5b4-d029dce539f0\"},{\"content\":{\"connectorIds\":[\"Out1\",\"Out2\",\"Out3\",\"Out4\",\"Out5\",\"Out6\",\"Out7\"],\"side\":\"RIGHT\"},\"type\":\"ConnectorPlacement.EquallySpacedRectSide\",\"uuid\":\"a61405db-f389-4151-925c-555d717cbde4\"},{\"content\":{\"side\":\"TOP\"},\"type\":\"ConnectorPlacement.EquallySpacedRectSide\",\"uuid\":\"de94411e-b629-424b-8cf2-091e2eaeef63\"},{\"content\":{\"connectorIds\":[\"In6\"],\"side\":\"BOTTOM\"},\"type\":\"ConnectorPlacement.EquallySpacedRectSide\",\"uuid\":\"bed50433-e632-4a1c-8813-e3713f42c747\"}]},\"type\":\"ConnectorPlacement.EquallySpacedConnector\",\"uuid\":\"788d2a2f-3ff0-43d4-a0ba-052de30f9400\"}],\"packageUris\":[\"http://schema.mathworks.com/mf0/Connector/R2020b\"],\"version\":\"1.0\"}"
  VI : Subsystem  mask{L=VI_L, R=VI_R, Tf=WOF_Tf}
      mask prompts: L "Inductance (pu)"; R "Resistance (pu)"; Tf "WOF time constant (s)"
      mask init: same as VFlexP_small/Grid/Dynamic/DCAC converters/DC_VCVSC/VI
  Voltage (pu) : Scope  NumInputPorts=2
      settings: ActiveDisplayYMinimum=0.67713076078540624  ActiveDisplayYMaximum=1.0454422045572083  DataLoggingVariableName=ScopeData9
  WOF_d : Subsystem
  Zero : Constant  Value=0  OutDataTypeStr=Inherit: Inherit via back propagation
  Zero1 : Constant  Value=0  OutDataTypeStr=Inherit: Inherit via back propagation
  connect : Subsystem
  frame : Integrator  InitialCondition=Grid_opDC_VSM.frame  IgnoreLimit=on
  iv : Integrator  InitialCondition=Grid_opDC_VSM.iv
  trim_output : Subsystem
  vod : Sum  Inputs=++|
  iac : Outport
  idc : Outport  Port=2
  tag scope: Pi_VSM=global, omega_DC_VSM=global
  wires:
  Sum8/1 -> VCC/2(voqref)
  vod/1 -> VCC/1(vodref)
  [omega] -> VI/3(omega)
  [ioq] -> VI/2(iq)
  [iod] -> VI/1(id)
  Gain2/1 -> Reference frame transform2/2(theta)
  [theta] -> Gain2/1
  PC/4(Q_f) -> [Q_s], [Q_f]
  PC/3(P_f) -> [P_s], [P_f]
  connect/3(connected) -> [connected]
  [omega] -> Sum2/2  "omega"
  [omega_ref] -> Sum2/1  "ref_omega"
  RL out/1(id) -> connect/1(id)
  [theta] -> Gain1/1
  Gain1/1 -> Reference frame transform1/2(theta)
  [ioq] -> VCC/4(ioq)
  [iod] -> VCC/3(iod)
  Zero/1 -> Sum8/2
  [vodref] -> vod/2
  [omega] -> VCC/5(omega)
  [theta] -> Reference frame transform3/2(theta)
  PC/1(omega) -> [omega_DC_VSM], [omega]
  PC/2(Out2) -> [vodref]
  [iod] -> PC/2(iodi)
  [ioq] -> PC/1(ioq)
  Reference frame transform1/2(out_q) -> [ioq]
  Reference frame transform3/1(out_d) -> RL out/1(v_in_d), Scope/1
  Reference frame transform3/2(out_q) -> RL out/3(v_in_q), Scope/2
  RL out/2(iq) -> connect/2(iq)
  Reference frame transform1/1(out_d) -> [iod]
  VI/1(vd) -> vod/1
  VI/2(vq) -> Sum8/1
  connect/1(id_real) -> trim_output/1(id), Matrix Concatenate1/1, Reference frame transform1/1(in_d)
  connect/2(iq_real) -> trim_output/2(iq), Matrix Concatenate1/2, Reference frame transform1/3(in_q)
  RL out/3(v_outd) -> Terminator1/1
  RL out/4(v_outq) -> Terminator2/1
  Reference frame transform2/1(out_d) -> LPF/1(In1)
  Reference frame transform2/2(out_q) -> LPF1/1(In1)
  [vqout] -> Reference frame transform2/3(in_q), Mux2/2, Reference frame transform4/2(in_q), Real-Imag to Complex/2, RL out/4(v_out_q)
  LPF/1(Out1) -> [v_d_PCC]
  LPF1/1(Out1) -> [v_q_PCC]
  [vdout] -> Reference frame transform4/1(in_d), Mux2/1, Real-Imag to Complex/1, RL out/2(v_out_d), Reference frame transform2/1(in_d)
  Matrix Concatenate1/1 -> Signal Specification1/1
  Constant/1 -> Matrix Concatenate1/3
  For Each Subsystem/1(Out1) -> iac/1
  Signal Specification1/1 -> For Each Subsystem/1(In1)
  [v_d_PCC] -> PC/5(vodi)
  [v_q_PCC] -> PC/6(voq)
  trim_output/1(Out1) -> Terminator/1
  trim_output/2(Out2) -> Terminator3/1
  trim_output/3(Out3) -> Terminator4/1
  trim_output/4(Out4) -> Terminator5/1
  vac/1 -> Selector6/1, Selector5/1
  Selector6/1 -> [vqout], trim_output/4(vq)
  Selector5/1 -> [vdout], trim_output/3(vd)
  VCC/1(vidref) -> [vod], Reference frame transform3/1(in_d)
  VCC/2(viqref) -> [voq], Reference frame transform3/3(in_q)
  Constant2/1 -> PC/7(Psp)
  Constant3/1 -> PC/8(Qsp)
  iv/1 -> Sum1/2
  One/1 -> connect/3(connect)
  Sum1/1 -> PC/4(Eref)
  vdc/1 -> Selector/1
  Transpose/1 -> State-Space/1
  Divide/1 -> Transpose/1  "iDC"
  Abs4/1 -> Product8/2, Product8/1, Gain3/1
  Transpose1/1 -> idc/1
  Product5/1 -> Sum4/2
  Product6/1 -> Sum6/3
  Sum4/1 -> [Pi_VSM], Sum6/2
  Sum5/1 -> Sum6/1
  State-Space/1 -> Transpose1/1
  Gain4/1 -> Sum5/1
  Gsw/1 -> Product6/1
  Real-Imag to Complex2/1 -> Abs4/1
  Constant1/1 -> Sum5/3
  Product4/1 -> Sum4/1
  Sum6/1 -> Gain10/1  "Pdc"
  Gain3/1 -> Sum5/2
  Gain10/1 -> Divide/1
  Product8/1 -> Gain4/1
  [viq] -> Product5/1
  Selector/1 -> Product6/3, Product6/2, [vDC], Divide/2
  [iiq] -> Product5/2, Real-Imag to Complex2/2  "ioq"
  [vid] -> Product4/1
  [iid] -> Product4/2, Real-Imag to Complex2/1  "iod"
  Gain7/1 -> frame/1
  VCC/3(iq_limited) -> [iq_limited]
  Sum2/1 -> Gain7/1
  VCC/4(iid) -> [iid]
  VCC/5(iiq) -> [iiq]
  VCC/6(vid) -> [vid]
  VCC/7(viq) -> [viq]
  One1/1 -> PC/3(omegaref), Sum1/1
  [vDC] -> Square/1
  Square/1 -> Sum3/1
  One2/1 -> Sum3/2
  frame/1 -> Sum7/1
  Sum7/1 -> [theta]
  Sum3/1 -> Dead Zone/1
  Gain6/1 -> Sum/1
  [Pi_VSM] -> Mux3/1, Active power (pu)/1, Mux1/1  "VFlexP"
  Gain5/1 -> Sum7/2
  [vDC] -> Square1/1
  Constant5/1 -> Sum11/2
  Step/1 -> Product/1
  [Pi_VSM] -> Sum14/2
  Step3/1 -> Sum9/2
  Sum14/1 -> Product/2
  Constant4/1 -> Sum9/1
  Sum9/1 -> Sum14/1
  Gain8/1 -> WOF_d/1(In1)
  Gain12/1 -> Sum12/1
  Sum11/1 -> Gain8/1, Gain12/1
  WOF_d/1(Out1) -> Sum12/2
  From File/1 -> Voltage (pu)/2, Mux/2  "Carlo"
  Gain14/1 -> Gain5/1
  Gain15/1 -> Gain6/1
  Sum16/1 -> Mux1/2, Mux3/2, Active power (pu)/2  "Carlo"
  Sum12/1 -> Gain11/1, LPF2/1(In1)
  Gain/1 -> LPF_1/1(In1)
  LPF2/1(Out1) -> Mux4/1, LPF_Pi/1
  [Pi_VSM] -> Sum10/1
  Sum10/1 -> LPF_Pi/2, Mux4/2
  Step1/1 -> Sum10/2
  Square1/1 -> Voltage (pu)/1, Mux/1, Sum11/1  "VFlexP"
  Mux/1 -> To Workspace/1
  Mux1/1 -> To File/1
  LPF_1/1(Out1) -> Sum/2
  Real-Imag to Complex/1 -> Complex to Magnitude-Angle/1
  Complex to Magnitude-Angle/2 -> Derivative/1
  [omega_ref] -> Sum13/1  "ref_omega"
  Sum13/1 -> Scope1/1
  Derivative/1 -> Gain16/1
  Gain16/1 -> Sum13/2
  PLL/1(Input2) -> Sum15/2, Integrator1/1  "omega2"
  Integrator1/1 -> Gain17/1
  Reference frame transform4/2(out_q) -> PLL/1(out_q)
  [omega_ref] -> Sum15/1  "ref_omega"
  Sum15/1 -> Scope2/1
  Gain17/1 -> Reference frame transform4/3(theta)
  [omega_ref] -> Gain18/1  "ref_omega"
  Integrator2/1 -> Inverse Park Transform/2
  Mux2/1 -> Inverse Park Transform/1
  Inverse Park Transform/1 -> Scope3/1
  Zero1/1 -> Mux2/3
  Gain18/1 -> Integrator2/1
  From File1/1 -> Sum16/1  "Carlo"
  Gain11/1 -> Gain/1, Gain15/1, Gain14/1
  Mux3/1 -> To Workspace1/1
  Mux4/1 -> To Workspace2/1
  Sum/1 -> PC/9(iomega)
